simulink model "pod_velocity_drag_SIM"  (R2020a)
settings: Solver=VariableStepAuto  StartTime=0.0  StopTime=10.0  RelTol=1e-3
values from neighbouring files (symbols this model uses):
  A = 21.927    [pod_velocity_drag.m]    (also in script_LIM.m = [3 5.8;4 5.189;5 4.62;6 4.1148;7 3.665;8 3.2639;9 2.9057;10 ; simulation_LIM.m = [3 5.8267)
  C0 = 0.05    [pod_velocity_drag.m]
  Cd = 0.193    [pod_velocity_drag.m]
  g = 9.81    [pod_velocity_drag.m]    (also in script_LIM.m = 1; simulation_LIM.m = 1; simulation_thrust.m = 0.01649)
  m = 81.7    [pod_velocity_drag.m]    (also in script_LIM.m = 3; simulation_LIM.m = 3)
  rho = 0.0097    [pod_velocity_drag.m]
settings Model: Creator=Bryan Poon  LastModifiedBy=Bryan Poon

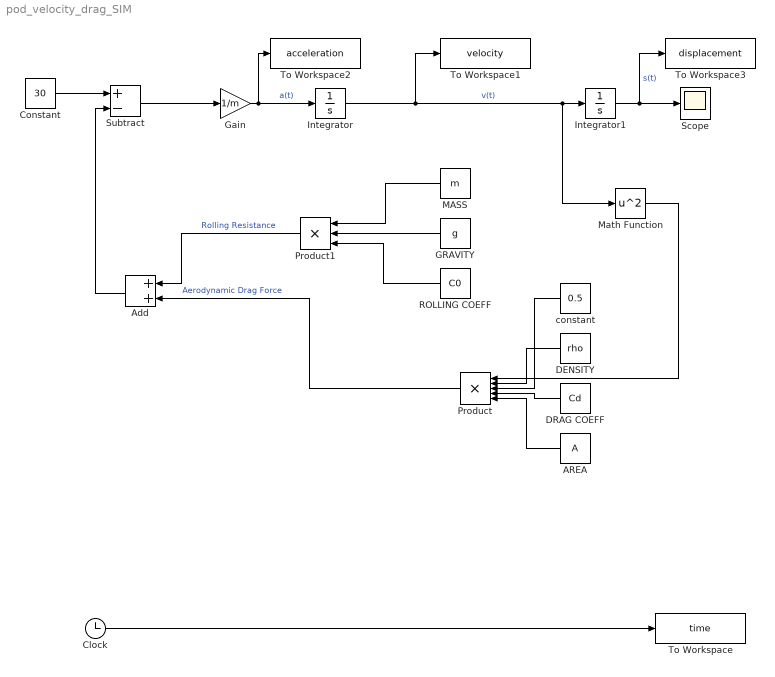
== system pod_velocity_drag_SIM ==
  AREA : Constant  Value=A
  Add : Sum
  Clock : Clock
  Constant : Constant  Value=30
  DENSITY : Constant  Value=rho
  DRAG COEFF : Constant  Value=Cd
  GRAVITY : Constant  Value=g
  Gain : Gain  Gain=1/m
  Integrator : Integrator
  Integrator1 : Integrator
  MASS : Constant  Value=m
  Math Function : Math  Operator=square  SaturateOnIntegerOverflow=on
  Product : Product  Inputs=5
  Product1 : Product  Inputs=3
  ROLLING COEFF : Constant  Value=C0
  Scope : Scope
  Subtract : Sum  Inputs=+-
  To Workspace : ToWorkspace  VariableName=time  SampleTime=-1
  To Workspace1 : ToWorkspace  VariableName=velocity  SampleTime=-1
  To Workspace2 : ToWorkspace  VariableName=acceleration  SampleTime=-1
  To Workspace3 : ToWorkspace  VariableName=displacement  SampleTime=-1
  constant : Constant  Value=0.5
  wires:
  Integrator1/1 -> To Workspace3/1, Scope/1  "s(t)"
  Integrator/1 -> To Workspace1/1, Math Function/1, Integrator1/1  "v(t)"
  DENSITY/1 -> Product/2
  DRAG COEFF/1 -> Product/4
  AREA/1 -> Product/5
  Product/1 -> Add/2  "Aerodynamic Drag Force"
  MASS/1 -> Product1/1
  GRAVITY/1 -> Product1/2
  ROLLING COEFF/1 -> Product1/3
  Product1/1 -> Add/1  "Rolling Resistance"
  Gain/1 -> To Workspace2/1, Integrator/1  "a(t)"
  Clock/1 -> To Workspace/1
  Add/1 -> Subtract/2
  Constant/1 -> Subtract/1
  Subtract/1 -> Gain/1
  Math Function/1 -> Product/1
  constant/1 -> Product/3
